simulink library "BrickPiSimLib"  (R2019a)
settings: Solver=VariableStepAuto  StartTime=0.0  StopTime=10.0  RelTol=1e-3
libraries: simulink x1, BrickPiSimSubLib_Read x1
settings Model: Creator=hahn  LastModifiedBy=uk008555

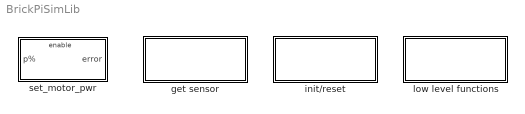
== system BrickPiSimLib ==
  get sensor : Subsystem
      settings: OpenFcn=BrickPiSimSubLib_getsensor
  init/reset : Subsystem
      settings: OpenFcn=BrickPiSimSubLib_initreset
  low level functions : Subsystem
      settings: OpenFcn=BrickPiSimSubLib_Read
  set_motor_pwr : Subsystem  StopFcn=""  mask{Add_Val=1, Port_Val=1}
      mask prompts: Add_Val "SPI Address"; Port_Val "Port"
      mask init:
      | port_val=Port_Val;
      | switch Port_Val
      |     case 1
      |         port_val='A';
      |     case 2
      |         port_val='B';
      |     case 3
      |         port_val='C';
      |     case 4
      |         port_val='D';
      |     otherwise
      |         port_val='failure';
      | end
      mask TypeOptions Add_Val: spi_writeRead_bpi/Add_Val
      mask TypeOptions Port_Val: spi_writeRead_bpi/Port_Val
      mask Display: disp(['Set\n MOTOR_PWR\n Motor: ' port_val])

== system BrickPiSimLib/get sensor ==

== system BrickPiSimLib/init//reset ==

== system BrickPiSimLib/low level functions ==

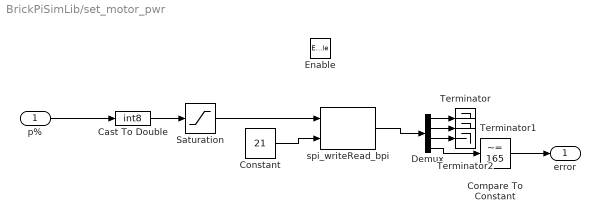
== system BrickPiSimLib/set_motor_pwr ==
  p% : Inport
  Enable : EnablePort
  Cast To Double : DataTypeConversion  OutDataTypeStr=int8
  Compare To Constant : simulink/Logic and Bit Operations/Compare To Constant  relop=~=  const=165  OutDataTypeStr=boolean
  Constant : Constant  Value=21  OutDataTypeStr=int8
  Demux : Demux
  Saturation : Saturate  UpperLimit=100  LowerLimit=-100  OutDataTypeStr=int8
  Terminator : Terminator
  Terminator1 : Terminator
  Terminator2 : Terminator
  spi_writeRead_bpi : BrickPiSimSubLib_Read/spi_writeRead_bpi  Add_Val=Add_Val  Port_Val=1
      settings: SourceProductName=Simulink Support Package for BrickPi
  error : Outport
  wires:
  Constant/1 -> spi_writeRead_bpi/2
  p%/1 -> Cast To Double/1
  spi_writeRead_bpi/1 -> Demux/1
  Saturation/1 -> spi_writeRead_bpi/1
  Demux/1 -> Terminator/1
  Demux/2 -> Terminator1/1
  Demux/3 -> Terminator2/1
  Demux/4 -> Compare To Constant/1
  Compare To Constant/1 -> error/1
  Cast To Double/1 -> Saturation/1
